simulink model "Asignacion1_grupo8"  (R2013a)
settings: Solver=ode45  StartTime=0.0  StopTime=10.0  RelTol=1e-3
settings Model: Creator=Edgar Maurette K  LastModifiedBy=Edgar Maurette K

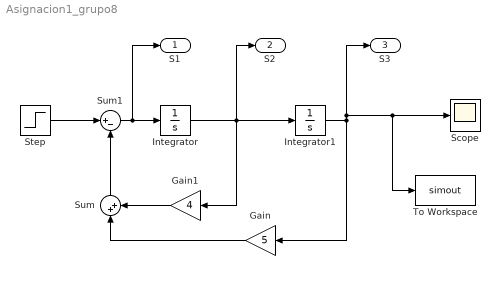
== system Asignacion1_grupo8 ==
  Gain : Gain  Gain=5
  Gain1 : Gain  Gain=4
  Integrator : Integrator
  Integrator1 : Integrator
  Scope : Scope
  Step : Step  SampleTime=0
  Sum : Sum  Inputs=|++
  Sum1 : Sum  Inputs=|+-
  To Workspace : ToWorkspace  VariableName=simout  SampleTime=-1  SaveFormat=Timeseries
  S1 : Outport
  S2 : Outport  Port=2
  S3 : Outport  Port=3
  wires:
  Integrator/1 -> S2/1, Gain1/1, Integrator1/1
  Integrator1/1 -> To Workspace/1, Scope/1, S3/1, Gain/1
  Sum1/1 -> S1/1, Integrator/1
  Gain1/1 -> Sum/2
  Sum/1 -> Sum1/2
  Gain/1 -> Sum/1
  Step/1 -> Sum1/1
